simulink model "reichardt_array_hyles_grating_osc"  (Simulink 9.2)
settings: Solver=ode45  StartTime=0.0  StopTime=setStopTime  FixedStep=0.0005  RelTol=1e-3  EnableMultiTasking=on
model workspace (MAT data in the model file):
  freq = 628.318530718
  headAmp = 4.5
  headPhase = 0
  outputTimeList = [1 1.0001 1.0002 1.0003 1.0004 1.0005 1.0006 1.0007 1.0008 1.0009 1.001 1.0011 1.0012 1.0013 1.0014 1.0015 1.0016 1.0017 1.0018 1.0019 1.002 1.0021 1.0022 1.0023 1.0024 1.0025 1.0026 1.0027 1.0028 1.0029 1.003 1.0031 1.0032 1.0033 1.0034 1.0035 1.0036 1.0037 1.0038 1.0039 1.004 1.0041 1.0042 1.0043 1.0044 1.0045 1.0046 1.0047 1.0048 1.0049 1.005 1.0051 1.0052 1.0053 1.0054 1.0055 1.0056 1.0057 1.0058 1.0059 1.006 1.0061 1.0062 1.0063 1.0064 1.0065 1.0066 1.0067 1.0068 1.0069 1.007 1.0071 1.0072 1.0073 1.0074 1.0075 1.0076 1.0077 1.0078 1.0079 1.008 1.0081 1.0082 1.0083 1.0084 1.0085 1.0086 1.0087 1.0088 1.0089 1.009 1.0091 1.0092 1.0093 1.0094 1.0095 1.0096 1.0097 1.0098 1.0099 1.01]
  setStopTime = 1.01
  stimAmp = 5
  temporalFilt = 0.046
  timeConstant = 0.046
values from neighbouring files (symbols this model uses):
  freq = freqData(jj,1).output(ii)    [EMD_sim.m]    (also in EMD_sim_v2.m; SS_fit_v2.m = 2*mean(diff(zx)); setup_reichardt_array_hyles_grating_osc.m = freqData(jj,kk).output(ii))
  temporalFilt = timeConstant    (= 0.046)    [run_simulink_model_grating_osc.m]
  timeConstant = 46e-3    (= 0.046)    [run_simulink_model_grating_osc.m]
libraries: visionsources x1
settings Model: LogicAnalyzerSignalOrdering=94723d94-0fb9-48a1-a8be-bee64210528d,a71c693a-e045-49f2-9a2b-fd1d6fda7f8e,6b902a21-b312-494c-94da-f4c8e853617c,db28250c-7404-4e50-ae35-76410c95bf8e,836d504f-1a60-4509-b72a-a4806fe259f8,c3d22241-23bf-4d79-9aab-67dc7151a41f  Creator=Shane  LastModifiedBy=BOC5244  SimulationMode=accelerator
settings DataIOCC: LimitDataPoints=off  SignalLoggingSaveFormat=Dataset  ReturnWorkspaceOutputs=on  OutputOption=SpecifiedOutputTimes  OutputTimes=outputTimeList
settings OptimizationCC: ExpressionDepthLimit=2147483647  EfficientMapNaN2IntZero=off  LifeSpan=auto  SimCompilerOptimization=on
settings HardwareCC: TargetBitPerPointer=64  TargetBitPerSizeT=64  TargetBitPerPtrDiffT=64  TargetLongLongMode=on  TargetIntDivRoundTo=Zero  TargetEndianess=LittleEndian  TargetWordSize=64  TargetHWDeviceType=MATLAB Host  ProdEqTarget=off
settings RTWCC: SystemTargetFile=accel.tlc  TemplateMakefile=accel_default_tmf  RTWVerbose=off  RTWUseLocalCustomCode=on
settings CodeAppCC: MaxIdLength=128  StateflowObjectComments=off
settings STFCustomTargetCC: ConcurrentExecutionCompliant=on  MATLABClassNameForMDSCustomization=Simulink.SoftwareTarget.TargetSpecificTriggerConfigurationBase  SystemTargetFile=accel.tlc

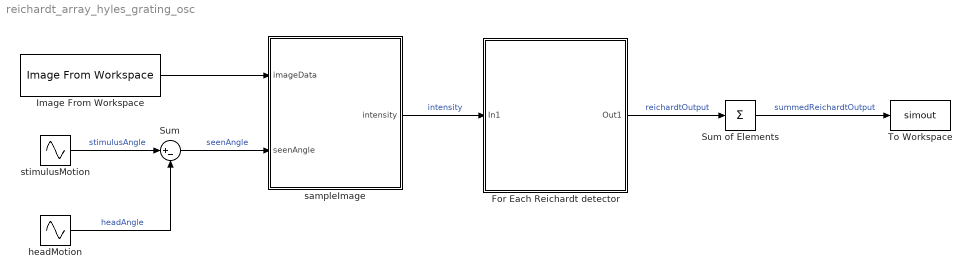
== system reichardt_array_hyles_grating_osc ==
  For Each Reichardt detector : Subsystem  TreatAsAtomicUnit=on
  Image From Workspace : visionsources/Image From Workspace  Tag=vipblks_nd  ImageValue=imageData  Ts=inf  imagePorts=One multidimensional signal  OutPortLabels=R|G|B  ImageDataType=double  Signed=on  WordLength=16  sdImageDataType=sfix(16)  FractionLengthMode=User-defined  FractionLength=15
      settings: SourceProductName=Computer Vision System Toolbox  SourceProductBaseCode=VP
  Sum : Sum  Inputs=|+-
  Sum of Elements : Sum  Inputs=+
  To Workspace : ToWorkspace  VariableName=simout  SaveFormat=Timeseries  SampleTime=-1
  headMotion : Sin  Amplitude=headAmp  Frequency=freq  Phase=headPhase  SampleTime=0
  sampleImage : MATLAB Function  TreatAsAtomicUnit=on
  stimulusMotion : Sin  Amplitude=stimAmp  Frequency=freq  SampleTime=0
  wires:
  For Each Reichardt detector/1(Out1) -> Sum of Elements/1  "reichardtOutput"
  Sum of Elements/1 -> To Workspace/1  "summedReichardtOutput"
  sampleImage/1(intensity) -> For Each Reichardt detector/1(In1)  "intensity"
  Image From Workspace/1 -> sampleImage/1(imageData)
  stimulusMotion/1 -> Sum/1  "stimulusAngle"
  headMotion/1 -> Sum/2  "headAngle"
  Sum/1 -> sampleImage/2(seenAngle)  "seenAngle"

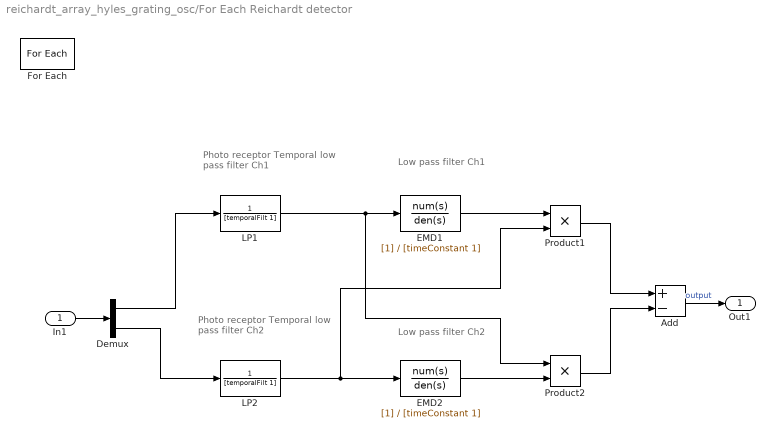
== system reichardt_array_hyles_grating_osc/For Each Reichardt detector ==
  note: Photo receptor
      | Temporal low pass filter
      | Ch2
  note: Photo receptor
      | Temporal low pass filter
      | Ch1
  note: Low pass filter
      | Ch1
  note: Low pass filter
      | Ch2
  In1 : Inport  Partition=on  PartitionDimension=1  PartitionWidth=1  PartitionOffset=0
  Add : Sum  Inputs=+-
  Demux : Demux  Outputs=2
  EMD1 : TransferFcn  Denominator=[timeConstant 1]
  EMD2 : TransferFcn  Denominator=[timeConstant 1]
  For Each : ForEach  DisableCoverage=on  IndexMode=One-based
  LP1 : TransferFcn  Numerator=1  Denominator=[temporalFilt 1]
  LP2 : TransferFcn  Numerator=1  Denominator=[temporalFilt 1]
  Product1 : Product  RndMeth=Zero
  Product2 : Product  RndMeth=Zero
  Out1 : Outport  ConcatenationDimension=1
  wires:
  EMD1/1 -> Product1/1
  Product1/1 -> Add/1
  Product2/1 -> Add/2
  EMD2/1 -> Product2/2
  Add/1 -> Out1/1  "output"
  Demux/1 -> LP1/1
  In1/1 -> Demux/1
  Demux/2 -> LP2/1
  LP2/1 -> EMD2/1, Product1/2
  LP1/1 -> EMD1/1, Product2/1

== matlab function sampleImage ==
  data: imageData input double; intensity output double size=360,2; seenAngle input double
function intensity = fcn(imageData,seenAngle)
%#codegen

imageWidth=length(imageData);

% subsample with resolution of compound eye
sampleCoord=0:359;
sampleCoord=sampleCoord+seenAngle;
sampleCoord=mod(sampleCoord,360);
temp=interp1(linspace(0,360,imageWidth),imageData,sampleCoord);

% create output signals
intensity=[temp(:), circshift(temp(:),-1)];
